simulink model "ZN_Stability_PI"  (R2018a)
settings: Solver=VariableStepAuto  StartTime=0.0  StopTime=300  RelTol=1e-3
values from neighbouring files (symbols this model uses):
  den_PI = [22.25 0]    [ZN_Stability.m]
  den_plant = conv([T1 1], conv([T2 1],[T3 1]))    [Classic_controller.m]    (also in Kessler_PID.m = conv([12.4 1], conv([5 1], [1.3 1])); ZN_Stability.m = conv([12.4 1], conv([5 1],[1.3 1])))
  num_PI = [51.73 2.325]    [ZN_Stability.m]
  num_plant = A    (= 1)    [Classic_controller.m]    (also in Kessler_PID.m; ZN_Stability.m)
  Tu = 3    [ZN_Stability.m]
settings Model: Creator=benko  LastModifiedBy=benko

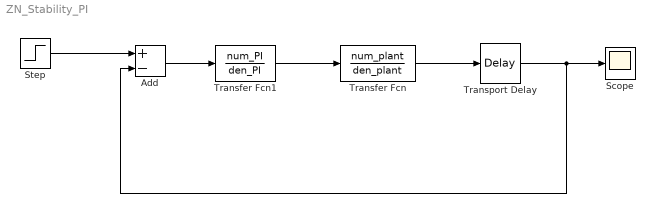
== system ZN_Stability_PI ==
  Add : Sum  Inputs=+-
  Scope : Scope
  Step : Step  SampleTime=0
  Transfer Fcn : TransferFcn  Numerator=num_plant  Denominator=den_plant
  Transfer Fcn1 : TransferFcn  Numerator=num_PI  Denominator=den_PI
  Transport Delay : TransportDelay  DelayTime=Tu
  wires:
  Transfer Fcn/1 -> Transport Delay/1
  Step/1 -> Add/1
  Transport Delay/1 -> Add/2, Scope/1
  Transfer Fcn1/1 -> Transfer Fcn/1
  Add/1 -> Transfer Fcn1/1
